simulink model "decoupleControl"  (R2024b)
settings: Solver=VariableStepAuto  StartTime=0.0  StopTime=1  RelTol=1e-3
undefined symbols (not defined in the file): A, B, C, F, K, r, x_0
settings Model: Creator=Longbin  LastModifiedBy=Longbin

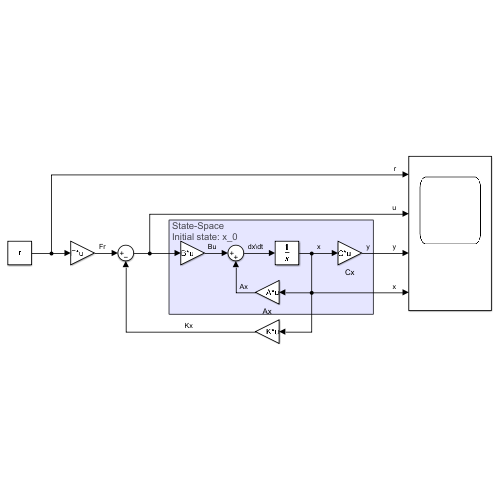
[thumbnail: Simulink's stored preview of the top-level diagram]
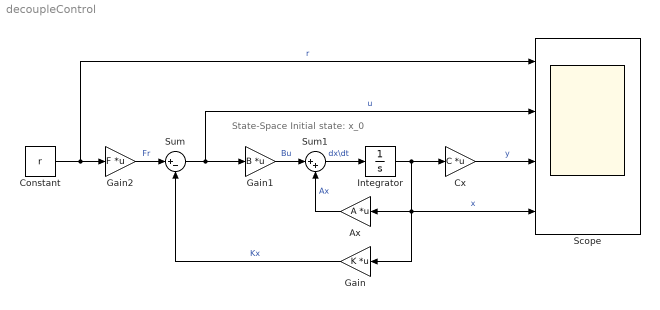
== system decoupleControl ==
  note: State-Space
      | Initial state: x_0
  Ax : Gain  Gain=A  Multiplication=Matrix(K*u)
  Constant : Constant  Value=r
  Cx : Gain  Gain=C  Multiplication=Matrix(K*u)
  Gain : Gain  Gain=K  Multiplication=Matrix(K*u)
  Gain1 : Gain  Gain=B  Multiplication=Matrix(K*u)
  Gain2 : Gain  Gain=F  Multiplication=Matrix(K*u)
  Integrator : Integrator  InitialCondition=x_0
  Scope : Scope  NumInputPorts=4
  Sum : Sum  Inputs=|+-
  Sum1 : Sum  Inputs=|++
  wires:
  Sum/1 -> Gain1/1, Scope/2  "u"
  Gain/1 -> Sum/2  "Kx"
  Ax/1 -> Sum1/2  "Ax"
  Gain1/1 -> Sum1/1  "Bu"
  Cx/1 -> Scope/3  "y"
  Sum1/1 -> Integrator/1  "dx\\dt"
  Integrator/1 -> Cx/1, Gain/1, Scope/4, Ax/1  "x"
  Constant/1 -> Gain2/1, Scope/1  "r"
  Gain2/1 -> Sum/1  "Fr"
